simulink model "continuous_time_vs"  (R2020b)
settings: Solver=ode45  StartTime=0.0  StopTime=10.0  MaxStep=0.5e-3  RelTol=1e-6
values from neighbouring files (symbols this model uses):
  e0 = s0 - C_features_desired(:)    [init.m]
  lambda = 10    [init.m]
undefined symbols (not defined in the file or in its folder): A__
settings Model: Creator=marco  LastModifiedBy=marco

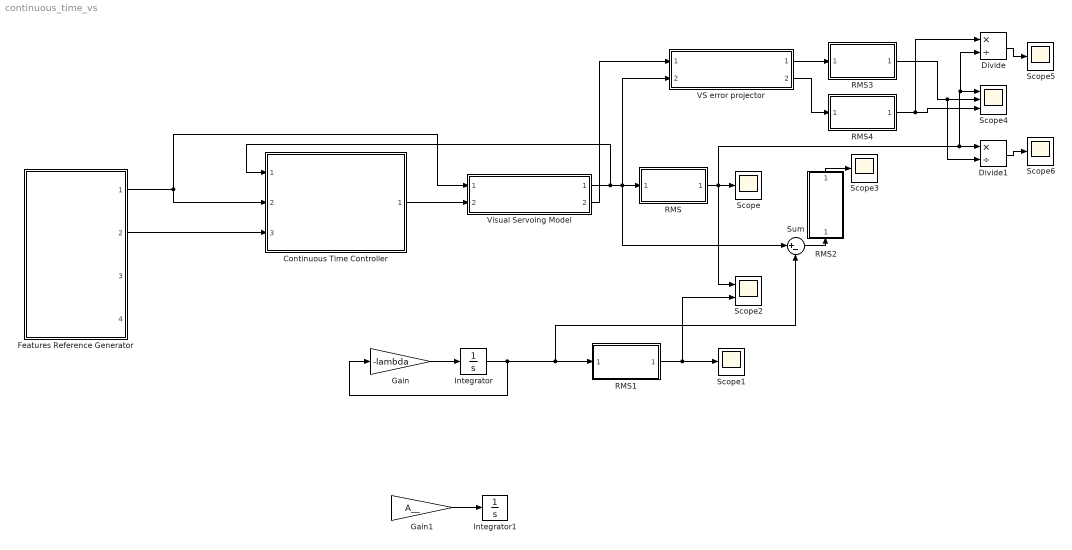
== system continuous_time_vs ==
  Continuous Time Controller : Subsystem  ReferencedSubsystem=continuous_time_controller  lambda=lambda  forward_action_enabled=off
  Divide : Product  Inputs=*/
  Divide1 : Product  Inputs=*/
  Features Reference Generator : Subsystem  ReferencedSubsystem=FeaturesReferenceGenerator  C_features_0=C_features_0  C_features_desired=C_features_desired  Cdesired_T_C0=Cdesired_T_C0.double  Ts=0  t0=0  tf=3  no_traj=on
  Gain : Gain  Gain=-lambda
  Gain1 : Gain  Gain=A__
  Integrator : Integrator  InitialCondition=e0
  Integrator1 : Integrator  InitialCondition=e0
  RMS{,1..4} (5 alike) : Subsystem  ReferencedSubsystem=RMS
  Scope{,1,3,5..6} (5 alike) : Scope
  Scope2 : Scope  NumInputPorts=2
  Scope4 : Scope  NumInputPorts=3
  Sum : Sum  Inputs=|+-
  VS error projector : Subsystem  ReferencedSubsystem=LProj
  Visual Servoing Model : Subsystem  ReferencedSubsystem=Features_System  s0=s0  noise_perc=0  noise_sample_time=0.1
  wires:
  Features Reference Generator/2 -> Continuous Time Controller/3
  Continuous Time Controller/1 -> Visual Servoing Model/2
  Visual Servoing Model/1 -> VS error projector/2, Sum/1, RMS/1, Continuous Time Controller/1
  RMS/1 -> Divide1/1, Divide/2, Scope4/1, Scope2/1, Scope/1
  Features Reference Generator/1 -> Continuous Time Controller/2, Visual Servoing Model/1
  Gain/1 -> Integrator/1
  Integrator/1 -> Sum/2, RMS1/1, Gain/1
  RMS1/1 -> Scope2/2, Scope1/1
  Sum/1 -> RMS2/1
  RMS2/1 -> Scope3/1
  Visual Servoing Model/2 -> VS error projector/1
  VS error projector/1 -> RMS3/1
  VS error projector/2 -> RMS4/1
  RMS4/1 -> Divide/1, Scope4/3
  Divide/1 -> Scope5/1
  RMS3/1 -> Divide1/2, Scope4/2
  Divide1/1 -> Scope6/1
  Gain1/1 -> Integrator1/1
